simulink model "M2V5_Motor_ParameterID_25a"  (R2025a)
settings: Solver=FixedStepDiscrete  StartTime=0.0  StopTime=inf  FixedStep=.004  RelTol=1e-3  EnableMultiTasking=on
libraries: arduinolib x2, simulink x1, arduinosensorlib x1
settings Model: SILPILModeSetting=veronly  ExtModeTrigDuration=2  Creator=hurstj  LastModifiedBy=hurstj
settings DataIOCC: SaveOutput=off  DSMLogging=off  SaveTime=off  ReturnWorkspaceOutputs=off
settings OptimizationCC: EnhancedBackFolding=on  PassReuseOutputArgsThreshold=0.0  MaxStackSize=64  OptimizeBlockOrder=speed  DifferentSizesBufferReuse=on  OptimizationCustomize=off
settings DebuggingCC: ParameterTunabilityLossMsg=error
settings HardwareCC: ProdBitPerInt=16.0  ProdBitPerPointer=16.0  ProdBitPerSizeT=16.0  ProdBitPerPtrDiffT=16.0  ProdLargestAtomicFloat=None  ProdWordSize=8.0  ProdHWDeviceType=Atmel->AVR  UseEmbeddedCoderFeatures=off  UseSimulinkCoderFeatures=off
settings ModelReferenceCC: EnableRefExpFcnMdlSchedulingChecks=on
settings SFSimCC: MATLABDynamicMemAlloc=off
settings RTWCC: SystemTargetFile=ert.tlc  HardwareBoard=Arduino Mega 2560  TemplateMakefile=ert_default_tmf  Toolchain=Arduino AVR  BuildConfiguration=Faster Runs  GPUComputeCapability=3.5  Description=Embedded Coder
settings CodeAppCC: ForceParamTrailComments=on  OperatorAnnotations=on
settings ERTTargetCC: ExtModeTransport=3.0  ExtModeStaticAllocSize=2048.0  InlinedParameterPlacement=Hierarchical  DynamicArrayContainerType=coder::array  ERTCustomFileBanners=off  SupportContinuousTime=on  SupportNonInlinedSFcns=on  RemoveResetFunc=off  SupportVariableSizeSignals=on  ModelStepFunctionPrototypeControlCompliant=off

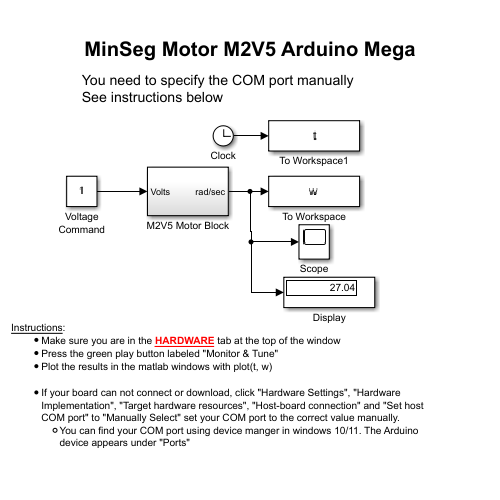
[thumbnail: Simulink's stored preview of the top-level diagram]
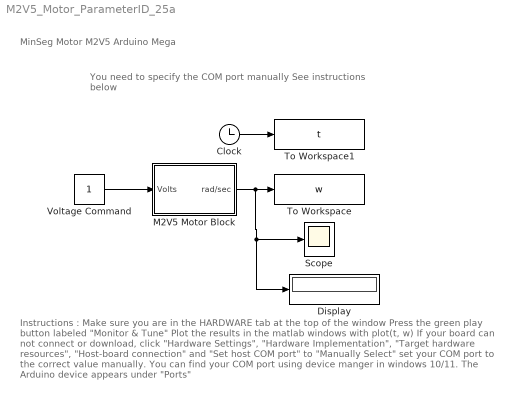
== system M2V5_Motor_ParameterID_25a ==
  note: Instructions :
      | Make sure you are in the HARDWARE tab at the top of the window
      | Press the green play button labeled "Monitor & Tune"
      | Plot the results in the matlab windows with plot(t, w)
      |
      | If your board can not connect or download, click "Hardware Settings", "Hardware Implementation", "Target hardware resources", "Host-board connection" and "Set host COM port" to "Manually Select" set your COM port to the correct value manually.
      | You can find your COM port using device manger in windows 10/11. The Arduino device appears under "Ports"
  note: You need to specify the COM port manually
      | See instructions below
  note: MinSeg Motor M2V5 Arduino Mega
  Clock : Clock
  Display : Display
  M2V5 Motor Block : Subsystem
  Scope : Scope
      settings: TimeSpan=30  ActiveDisplayYMinimum=-28.2179  ActiveDisplayYMaximum=253.96108  DataLoggingSaveFormat=Array
  To Workspace : ToWorkspace  VariableName=w  SampleTime=-1
      settings: Save2DSignal=2-D array (concatenate along first dimension)
  To Workspace1 : ToWorkspace  VariableName=t  SampleTime=-1
      settings: Save2DSignal=2-D array (concatenate along first dimension)
  Voltage Command : Constant
  wires:
  M2V5 Motor Block/1(rad/sec) -> Display/1, Scope/1, To Workspace/1
  Clock/1 -> To Workspace1/1
  Voltage Command/1 -> M2V5 Motor Block/1(Volts)

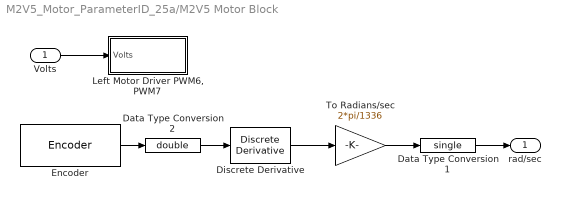
== system M2V5_Motor_ParameterID_25a/M2V5 Motor Block ==
  Volts : Inport
  Data Type Conversion1 : DataTypeConversion  OutDataTypeStr=single  SaturateOnIntegerOverflow=off  RndMeth=Floor
  Data Type Conversion2 : DataTypeConversion  OutDataTypeStr=double  SaturateOnIntegerOverflow=off  RndMeth=Floor
  Discrete Derivative : simulink/Discrete/Discrete Derivative  gainval=1.0  ICPrevScaledInput=0.0  OutMin=[]  OutMax=[]  OutDataType=fixdt(1, 16)  OutScaling=2^-10  DoSatur=off
  Encoder : arduinosensorlib/Encoder  InputA=2  InputB=3  Mode=No reset  SampleTime=-1
  "Left Motor Driver PWM6, PWM7" : Subsystem  mask{Vsupply=4.7, Voffset=0}
      mask prompts: Vsupply "Driver Voltage"; Voffset "Voltage offset (0-Vsupply)"
      mask help:
      | Specify driver supply voltage (3.9 for USB)
      | Specify the PWM offset (0-255)
      mask Display:
      | port_label('input',1,'Volts')
      | text(15,5,['Vsupply=' num2str(Vsupply)])
  To Radians/sec : Gain  Gain=2*pi/1336
  rad/sec : Outport
  wires:
  Discrete Derivative/1 -> To Radians/sec/1
  To Radians/sec/1 -> Data Type Conversion1/1
  Encoder/1 -> Data Type Conversion2/1
  Data Type Conversion2/1 -> Discrete Derivative/1
  Data Type Conversion1/1 -> rad/sec/1
  Volts/1 -> "Left Motor Driver PWM6, PWM7"/1(Volts)

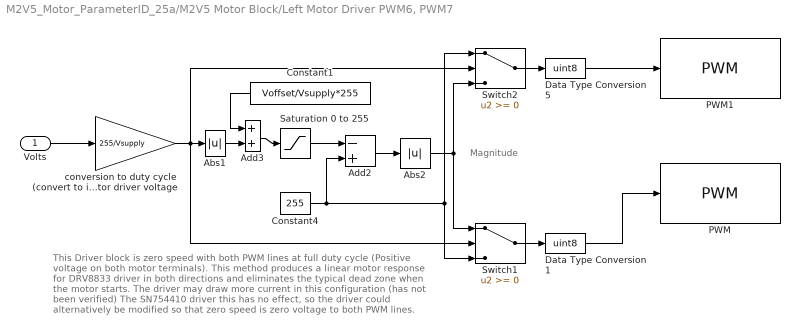
== system M2V5_Motor_ParameterID_25a/M2V5 Motor Block/Left Motor Driver PWM6, PWM7 ==
  note: Magnitude
  note: This Driver block is zero speed with both PWM lines at full duty cycle
      |  (Positive voltage on both motor terminals).
      | This method produces a linear motor response for DRV8833 driver
      |  in both directions and eliminates
      | the typical dead zone when the motor starts.
      | The driver may draw more current in this configuration (has not been verified)
      |
      | The SN754410 driver this has no effect, so the driver could alternatively
      | be modified so that zero speed is zero voltage to both PWM lines.
  Volts : Inport
  Abs1 : Abs  SaturateOnIntegerOverflow=off
  Abs2 : Abs  SaturateOnIntegerOverflow=off
  Add2 : Sum  Inputs=-+
  Add3 : Sum
  Constant1 : Constant  Value=Voffset/Vsupply*255
  Constant4 : Constant  Value=255
  Data Type Conversion1 : DataTypeConversion  OutDataTypeStr=uint8  SaturateOnIntegerOverflow=off  RndMeth=Floor
  Data Type Conversion5 : DataTypeConversion  OutDataTypeStr=uint8  SaturateOnIntegerOverflow=off  RndMeth=Floor
  PWM : arduinolib/PWM  pinNumber=7  frequencyType=Specify  desiredFrequency=32000  achievableFrequency=32000
  PWM1 : arduinolib/PWM  pinNumber=6  frequencyType=Specify  desiredFrequency=32000  achievableFrequency=32000
  Saturation 0 to 255 : Saturate  UpperLimit=255  LowerLimit=0
  Switch1 : Switch  SaturateOnIntegerOverflow=off  InputSameDT=off
  Switch2 : Switch  SaturateOnIntegerOverflow=off  InputSameDT=off
  conversion to duty cycle (convert to int) denominator is motor driver voltage : Gain  Gain=255/Vsupply  OutDataTypeStr=int16
  wires:
  Data Type Conversion1/1 -> PWM/1
  Data Type Conversion5/1 -> PWM1/1
  Switch1/1 -> Data Type Conversion1/1
  Switch2/1 -> Data Type Conversion5/1
  Abs2/1 -> Switch1/1, Switch2/3
  Add2/1 -> Abs2/1
  Constant4/1 -> Add2/2, Switch2/1, Switch1/3
  Saturation 0 to 255/1 -> Add2/1
  conversion to duty cycle (convert to int) denominator is motor driver voltage/1 -> Abs1/1, Switch2/2, Switch1/2
  Abs1/1 -> Add3/2
  Constant1/1 -> Add3/1
  Add3/1 -> Saturation 0 to 255/1
  Volts/1 -> conversion to duty cycle (convert to int) denominator is motor driver voltage/1
